simulink model "PhaseAngle_TestModel"  (R2014a)
settings: Solver=ode45  StartTime=0.0  StopTime=10.0  RelTol=1e-3
libraries: rocket_angular_flight_library x1
settings Model: Creator=scorpii  LastModifiedBy=scorpii

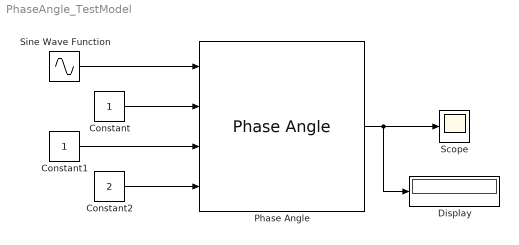
== system PhaseAngle_TestModel ==
  Constant : Constant
  Constant1 : Constant
  Constant2 : Constant  Value=2
  Display : Display
  Phase Angle : rocket_angular_flight_library/Phase Angle
  Scope : Scope
  Sine Wave Function : Sin  SampleTime=0
  wires:
  Sine Wave Function/1 -> Phase Angle/1
  Constant/1 -> Phase Angle/2
  Constant1/1 -> Phase Angle/3
  Constant2/1 -> Phase Angle/4
  Phase Angle/1 -> Display/1, Scope/1
